simulink model "ZumoSimulatiom_Path_Control"  (R2022b)
settings: Solver=ode15s  StartTime=0.0  StopTime=60  RelTol=1e-3
PreLoadFcn:
  | InitZumo
InitFcn:
  | InitZumo
values from neighbouring files (symbols this model uses):
  a_Max = 1/4    (= 0.25)    [InitZumo.m]
  GearRatio = 75    [InitZumo.m]
  Phi_Init = 0    [InitZumo.m]
  Robot_L = 98/1000    (= 0.098)    [InitZumo.m]
  sampleTime = 0.01    [InitZumo.m]
  v_Max = 1/2    (= 0.5)    [InitZumo.m]
  WheelRadius = 37.5/2/1000    (= 0.01875)    [InitZumo.m]
  X_Pos_Init = 0    [InitZumo.m]
  Y_Pos_Init = 0    [InitZumo.m]
libraries: fl_lib x32, nesl_utility x16, ee_lib x8, sdl_lib x2, slpidlib x2, simulink_extras x2
(part 2 of 2)

== matlab function ZumoSimulatiom_Path_Control/Path Control ==
  data: DesiredPos input; CurrPos input; V_Forward output; PHI input; theta_t output; de output; dist output; a_Max input; En output
function [V_Forward, theta_t, de, dist, En] = P2P_CTRL(DesiredPos,CurrPos,PHI,a_Max)

persistent currPoint
if isempty(currPoint)
    currPoint = 1;
end
% define the stopping distance and the pass to next point distance in [m]
stopDistance = 0.01;
passDistance = 0.05;

% number of desired points
numPoints = size(DesiredPos,1);

% calculate car vectors and Path vectors
Vr = [cos(PHI) , sin(PHI)]; % car direction vector
Vt = DesiredPos(currPoint,:)-CurrPos'; % car direction vector
% calculate alog which vector to move and to which point to reach

if (currPoint <= numPoints) && (currPoint > 1)
    Vd = DesiredPos(currPoint,:) - DesiredPos(currPoint-1,:);
else
    Vd = DesiredPos(currPoint,:) - [0 0]; % initial condition
end

crossVdVr = Vd(2)*Vr(1) - Vd(1)*Vr(2);  % cross(Vr,Vd)
crossVtVd =  Vt(2)*Vd(1) - Vt(1)*Vd(2); % cross(Vr,Vd)
dotVdVr = (Vd*Vr')/(norm(Vd)*norm(Vr)); % dot(vd,vr)

de = crossVtVd / norm(Vd); % distance to desired path

% claculate distance
dist = norm(Vt); % distance to current point
pathDist = 0; % remaining points distance

% sum of remaining points
if (currPoint < numPoints)
    for i = (currPoint):(numPoints-1)
        pathDist = pathDist + sqrt(sum((DesiredPos(i+1,:)-DesiredPos(i,:)).^2)); % sum of the distances of the rest of the points
    end
    % pass to next point condition
    if (abs(dist) < passDistance)
        currPoint = currPoint + 1;
    else % check if for some reason we missed the point. may cause to skip points
        dist_nextPoint = norm(DesiredPos(currPoint+1,:)-CurrPos');
        if (dist_nextPoint < dist) 
            currPoint = currPoint + 1;
        end
    end
    % update remaining distance
    dist = dist + pathDist;
end

% calculate the desired angle change for the target point
if (abs(crossVdVr) < 0.001) % Math singularity
    if (dotVdVr == -1) % vectors align in reverse... singularity
        theta_t = pi/2;
    else  % Vectors align in the same direction
        theta_t = 0;
    end
else
    dir = sign(crossVdVr);
    theta_t = acos(dotVdVr) * dir; % angle from desired path
end


% set desired velocity
if (currPoint == numPoints) % stop condition, happens only if reached last point
    if ((abs(dist) < stopDistance) || ((Vt*Vr')/norm(Vr) < -0.1)) % delta(d) - in case we missed the last point
        V_Forward = 0;
        theta_t = 0;
        En= 0;
    else
        V_Forward  = sqrt(2*a_Max*dist); % set desired velocity
        En = 1;
    end
else
    V_Forward  = sqrt(2*a_Max*dist);
    En = 1;
end

end
